simulink model "mrefrobotarm_modified_previous_y_previous_u_previous_ref_pert"  (R2018b)
settings: Solver=FixedStepAuto  StartTime=0.0  StopTime=10  RelTol=1e-3  AbsTol=1e-6
undefined symbols (not defined in the file or in its folder): cc, options
libraries: neural x714, simulink x1
(part 20 of 26)

== system mrefrobotarm_modified_previous_y_previous_u_previous_ref_pert/sd=0.1/Layer 3/Delays 1 ==
  "p{3}" : Inport  PortDimensions=30
      mask Display: e = 0.06;c1 = [120 230 180]/255;c2 = ([120 230 180]+0)/(256+128);c3 = ([120 230 180]+128)/(256+128);patch([0 1 1 0],[0 0 1 1],c1);patch([0 1 1 1-e 1-e 0+e],[0 0 1 1-e 0+e 0+e],c2);patch([0 0 1 1-e 0+e 0+e],[0 1 1 1-e 1-e 0+e],c3);plot([0 1 1 0 0],[0 0 1 1 0]);
  mux : Mux  Inputs=1
      mask Display: e = 0.06;c1 = [120 150 230]/255;c2 = ([120 150 230]+0)/383;c3 = ([120 150 230]+128)/383;patch([0 1 1 0],[0 0 1 1],c1);patch([0 1 1 1-e 1-e 0+e],[0 0 1 1-e 0+e 0+e],c2);patch([0 0 1 1-e 0+e 0+e],[0 1 1 1-e 1-e 0+e],c3);plot([0 1 1 0 0],[0 0 1 1 0]);disp('Mux')
  "pd{3,2}" : Outport
      mask Display: e = 0.06;c1 = [120 230 180]/255;c2 = ([120 230 180]+0)/(256+128);c3 = ([120 230 180]+128)/(256+128);patch([0 1 1 0],[0 0 1 1],c1);patch([0 1 1 1-e 1-e 0+e],[0 0 1 1-e 0+e 0+e],c2);patch([0 0 1 1-e 0+e 0+e],[0 1 1 1-e 1-e 0+e],c3);plot([0 1 1 0 0],[0 0 1 1 0]);
  wires:
  "p{3}"/1 -> mux/1
  mux/1 -> "pd{3,2}"/1

== system mrefrobotarm_modified_previous_y_previous_u_previous_ref_pert/sd=0.1/Layer 3/LW{3,2} ==
  "ad{3,2}" : Inport  PortDimensions=30
      mask Display: e = 0.06;c1 = [120 230 180]/255;c2 = ([120 230 180]+0)/(256+128);c3 = ([120 230 180]+128)/(256+128);patch([0 1 1 0],[0 0 1 1],c1);patch([0 1 1 1-e 1-e 0+e],[0 0 1 1-e 0+e 0+e],c2);patch([0 0 1 1-e 0+e 0+e],[0 1 1 1-e 1-e 0+e],c3);plot([0 1 1 0 0],[0 0 1 1 0]);
  "IW{3,2}(1,:)'" : Constant  Value=[0.0018188839666211098489156938740052282810211181640625;-0.0126510816907239136142049318323188344947993755340576171875;-0.00597472431956966830435273863031397922895848751068115234375;0.005949992205404812384283985693400609306991100311279296875;-0.018958893167521397027375229527024202980101108551025390625;-0.007711057222642365809039954882564416038803756237030029296875;-0.010778308261510882726241788986953906714916229248046875;0.054764058581412124182552503270926536060869693756103515625;0.006862056331544587849113892019659033394418656826019287109375;0.00715707547253511232321354640362187637947499752044677734375;-0.0016983245624861524614157559653904172591865062713623046875;-0.0065973873363838371475242894348411937244236469268798828125;-0.037341973875675053828881999606892350129783153533935546875;0.0018086616996149107450264637009240686893463134765625;-0.00260391987922085899054280844211461953818798065185546875;-0.0307949849301379675881040753893103101290762424468994140625;0.0170954132041403715491778569912639795802533626556396484375;-0.00466213820726418988471539961437883903272449970245361328125;0.004629973795378283969725874413825295050628483295440673828125;-0.0119610632763333425698792922275970340706408023834228515625;-0.01430710633569359270522713956097504706121981143951416015625;-0.033746901411126815906182940807411796413362026214599609375;0.50788162427434002665904699824750423431396484375;0.0104845825353180772954164723387293634004890918731689453125;-0.0039154731651121210678212491984595544636249542236328125;0.00908007893074675755118452258329853066243231296539306640625;0.004049068749268728943657702501468520495109260082244873046875;-0.0007508777613577442659742455788318693521432578563690185546875;-0.002722985317096936197511780619606724940240383148193359375;0.002330981056152135223735744062878438853658735752105712890625]
      mask Display: e = 0.06;c1 = [120 150 230]/255;c2 = ([120 150 230]+0)/383;c3 = ([120 150 230]+128)/383;patch([0 1 1 0],[0 0 1 1],c1);patch([0 1 1 1-e 1-e 0+e],[0 0 1 1-e 0+e 0+e],c2);patch([0 0 1 1-e 0+e 0+e],[0 1 1 1-e 1-e 0+e],c3);plot([0 1 1 0 0],[0 0 1 1 0]);disp('weights');
  Mux : Mux  Inputs=1
      mask Display: e = 0.06;c1 = [120 150 230]/255;c2 = ([120 150 230]+0)/383;c3 = ([120 150 230]+128)/383;patch([0 1 1 0],[0 0 1 1],c1);patch([0 1 1 1-e 1-e 0+e],[0 0 1 1-e 0+e 0+e],c2);patch([0 0 1 1-e 0+e 0+e],[0 1 1 1-e 1-e 0+e],c3);plot([0 1 1 0 0],[0 0 1 1 0]);disp('Mux');
  dotprod1 : neural/Weight Functions/dotprod
  "lz{3,2}" : Outport
      mask Display: e = 0.06;c1 = [120 230 180]/255;c2 = ([120 230 180]+0)/(256+128);c3 = ([120 230 180]+128)/(256+128);patch([0 1 1 0],[0 0 1 1],c1);patch([0 1 1 1-e 1-e 0+e],[0 0 1 1-e 0+e 0+e],c2);patch([0 0 1 1-e 0+e 0+e],[0 1 1 1-e 1-e 0+e],c3);plot([0 1 1 0 0],[0 0 1 1 0]);
  wires:
  "IW{3,2}(1,:)'"/1 -> dotprod1/1
  "ad{3,2}"/1 -> dotprod1/2
  dotprod1/1 -> Mux/1
  Mux/1 -> "lz{3,2}"/1

== system mrefrobotarm_modified_previous_y_previous_u_previous_ref_pert/sd=0.2/Layer 1/Delays 1 ==
  "p{1}" : Inport  PortDimensions=10
      mask Display: e = 0.06;c1 = [120 230 180]/255;c2 = ([120 230 180]+0)/(256+128);c3 = ([120 230 180]+128)/(256+128);patch([0 1 1 0],[0 0 1 1],c1);patch([0 1 1 1-e 1-e 0+e],[0 0 1 1-e 0+e 0+e],c2);patch([0 0 1 1-e 0+e 0+e],[0 1 1 1-e 1-e 0+e],c3);plot([0 1 1 0 0],[0 0 1 1 0]);
  mux : Mux  Inputs=1
      mask Display: e = 0.06;c1 = [120 150 230]/255;c2 = ([120 150 230]+0)/383;c3 = ([120 150 230]+128)/383;patch([0 1 1 0],[0 0 1 1],c1);patch([0 1 1 1-e 1-e 0+e],[0 0 1 1-e 0+e 0+e],c2);patch([0 0 1 1-e 0+e 0+e],[0 1 1 1-e 1-e 0+e],c3);plot([0 1 1 0 0],[0 0 1 1 0]);disp('Mux')
  "pd{1,1}" : Outport
      mask Display: e = 0.06;c1 = [120 230 180]/255;c2 = ([120 230 180]+0)/(256+128);c3 = ([120 230 180]+128)/(256+128);patch([0 1 1 0],[0 0 1 1],c1);patch([0 1 1 1-e 1-e 0+e],[0 0 1 1-e 0+e 0+e],c2);patch([0 0 1 1-e 0+e 0+e],[0 1 1 1-e 1-e 0+e],c3);plot([0 1 1 0 0],[0 0 1 1 0]);
  wires:
  "p{1}"/1 -> mux/1
  mux/1 -> "pd{1,1}"/1

== system mrefrobotarm_modified_previous_y_previous_u_previous_ref_pert/sd=0.2/Layer 1/IW{1,1} ==
  "pd{1,1}" : Inport  PortDimensions=10
      mask Display: e = 0.06;c1 = [120 230 180]/255;c2 = ([120 230 180]+0)/(256+128);c3 = ([120 230 180]+128)/(256+128);patch([0 1 1 0],[0 0 1 1],c1);patch([0 1 1 1-e 1-e 0+e],[0 0 1 1-e 0+e 0+e],c2);patch([0 0 1 1-e 0+e 0+e],[0 1 1 1-e 1-e 0+e],c3);plot([0 1 1 0 0],[0 0 1 1 0]);
  "IW{1,1}(1,:)'" : Constant  Value=[0.51497279749678614990671121631748974323272705078125;1.206829650462811986955102838692255318164825439453125;-0.0843780927922921641926023994528804905712604522705078125;1.0983052451279047279086853450280614197254180908203125;1.826296411118257356775984590058214962482452392578125;-0.229783480998378475401722198512288741767406463623046875;0.44712104438269906214742377414950169622898101806640625;-0.342730536328451018679430717384093441069126129150390625;1.0259047401059024906544436817057430744171142578125;-0.2128168709740031749877431366257951594889163970947265625]
      mask Display: e = 0.06;c1 = [120 150 230]/255;c2 = ([120 150 230]+0)/383;c3 = ([120 150 230]+128)/383;patch([0 1 1 0],[0 0 1 1],c1);patch([0 1 1 1-e 1-e 0+e],[0 0 1 1-e 0+e 0+e],c2);patch([0 0 1 1-e 0+e 0+e],[0 1 1 1-e 1-e 0+e],c3);plot([0 1 1 0 0],[0 0 1 1 0]);disp('Weights');
  "IW{1,1}(10,:)'" : Constant  Value=[-0.290019837810844283154665390611626207828521728515625;1.202814314763049008405459971982054412364959716796875;0.64575006256269118498636316871852613985538482666015625;0.51228702422282612616299957153387367725372314453125;0.53897724154057058409961200595716945827007293701171875;0.2169804329551216770521904209090280346572399139404296875;1.109828612580184170610664295963943004608154296875;0.62047060970846767968822632610681466758251190185546875;0.701249951108816826916836362215690314769744873046875;-0.2409479446688067849624559357835096307098865509033203125]
      mask Display: e = 0.06;c1 = [120 150 230]/255;c2 = ([120 150 230]+0)/383;c3 = ([120 150 230]+128)/383;patch([0 1 1 0],[0 0 1 1],c1);patch([0 1 1 1-e 1-e 0+e],[0 0 1 1-e 0+e 0+e],c2);patch([0 0 1 1-e 0+e 0+e],[0 1 1 1-e 1-e 0+e],c3);plot([0 1 1 0 0],[0 0 1 1 0]);disp('Weights');
  "IW{1,1}(11,:)'" : Constant  Value=[-0.483965255554764939294187797713675536215305328369140625;-0.00423735713268407789000580265792450518347322940826416015625;-0.04071278147423264270887699467493803240358829498291015625;-0.063810707355427875864251063831034116446971893310546875;0.63945678291134344650714638191857375204563140869140625;-0.293214326660526103385251417421386577188968658447265625;-0.2489985904371469771501068635188858024775981903076171875;-0.243620889480985258757073097513057291507720947265625;0.89874278529941487025922697284840978682041168212890625;0.391843733467475308085425922399736009538173675537109375]
      mask Display: e = 0.06;c1 = [120 150 230]/255;c2 = ([120 150 230]+0)/383;c3 = ([120 150 230]+128)/383;patch([0 1 1 0],[0 0 1 1],c1);patch([0 1 1 1-e 1-e 0+e],[0 0 1 1-e 0+e 0+e],c2);patch([0 0 1 1-e 0+e 0+e],[0 1 1 1-e 1-e 0+e],c3);plot([0 1 1 0 0],[0 0 1 1 0]);disp('Weights');
  "IW{1,1}(12,:)'" : Constant  Value=[0.1612342900655281130450902082884567789733409881591796875;0.83783524521083052594150331060518510639667510986328125;-0.6105547643586188844011530818534083664417266845703125;0.93437549886920745478846583864651620388031005859375;-0.41271403386041505267911588816787116229534149169921875;-0.2038648125981606662460166035089059732854366302490234375;-0.79779908968110169187326619066880084574222564697265625;0.212892509754028680379889237883617170155048370361328125;1.613792336196116838920033842441625893115997314453125;-0.005932794346736929014252126535211573354899883270263671875]
      mask Display: e = 0.06;c1 = [120 150 230]/255;c2 = ([120 150 230]+0)/383;c3 = ([120 150 230]+128)/383;patch([0 1 1 0],[0 0 1 1],c1);patch([0 1 1 1-e 1-e 0+e],[0 0 1 1-e 0+e 0+e],c2);patch([0 0 1 1-e 0+e 0+e],[0 1 1 1-e 1-e 0+e],c3);plot([0 1 1 0 0],[0 0 1 1 0]);disp('Weights');
  "IW{1,1}(13,:)'" : Constant  Value=[-0.1362341877538358059229750551821780391037464141845703125;0.954572016628826958140052738599479198455810546875;1.4567774435177611724867574594100005924701690673828125;0.1398942982446665095341842288689804263412952423095703125;0.22521814577160992332238720337045378983020782470703125;0.94253660172752018464592538293800316751003265380859375;0.6447180725726564531896656262688338756561279296875;0.782760397215020109484839849756099283695220947265625;-0.755379723776314460081948709557764232158660888671875;0.7209229108371120187115366206853650510311126708984375]
      mask Display: e = 0.06;c1 = [120 150 230]/255;c2 = ([120 150 230]+0)/383;c3 = ([120 150 230]+128)/383;patch([0 1 1 0],[0 0 1 1],c1);patch([0 1 1 1-e 1-e 0+e],[0 0 1 1-e 0+e 0+e],c2);patch([0 0 1 1-e 0+e 0+e],[0 1 1 1-e 1-e 0+e],c3);plot([0 1 1 0 0],[0 0 1 1 0]);disp('Weights');
  "IW{1,1}(14,:)'" : Constant  Value=[0.3848296502569208410449164148303680121898651123046875;-0.0848479163709470185494865290820598602294921875;-0.06685187407183122709763978264163597486913204193115234375;-0.12513880958835532641870713632670231163501739501953125;0.803549161421274416028381892829202115535736083984375;-1.130139231574783575950959857436828315258026123046875;-0.191640285152762268605641793328686617314815521240234375;0.212885117495971110113117674700333736836910247802734375;1.0074860578633748620092092096456326544284820556640625;-0.5140243939426916153223601213539950549602508544921875]
      mask Display: e = 0.06;c1 = [120 150 230]/255;c2 = ([120 150 230]+0)/383;c3 = ([120 150 230]+128)/383;patch([0 1 1 0],[0 0 1 1],c1);patch([0 1 1 1-e 1-e 0+e],[0 0 1 1-e 0+e 0+e],c2);patch([0 0 1 1-e 0+e 0+e],[0 1 1 1-e 1-e 0+e],c3);plot([0 1 1 0 0],[0 0 1 1 0]);disp('Weights');
  "IW{1,1}(15,:)'" : Constant  Value=[0.50448118661232588255671771548804827034473419189453125;0.75534739506285131227514284546487033367156982421875;0.7186274496868938488347566817537881433963775634765625;1.1053410499284714862966438886360265314579010009765625;1.55113744248226215205477274139411747455596923828125;-0.84818341679632347496209376913611777126789093017578125;0.85626822715970429822363030325504951179027557373046875;1.0587139812572943231572253353078849613666534423828125;-1.3036773470877511815757543445215560495853424072265625;-0.2345687264122083004469487832466256804764270782470703125]
      mask Display: e = 0.06;c1 = [120 150 230]/255;c2 = ([120 150 230]+0)/383;c3 = ([120 150 230]+128)/383;patch([0 1 1 0],[0 0 1 1],c1);patch([0 1 1 1-e 1-e 0+e],[0 0 1 1-e 0+e 0+e],c2);patch([0 0 1 1-e 0+e 0+e],[0 1 1 1-e 1-e 0+e],c3);plot([0 1 1 0 0],[0 0 1 1 0]);disp('Weights');
  "IW{1,1}(16,:)'" : Constant  Value=[0.89365107384404296464452954751322977244853973388671875;-0.5783582377704370447446535763447172939777374267578125;0.420643159623975193550649009921471588313579559326171875;0.71330291898780273651681227420340292155742645263671875;-0.1639046914328597670529319429988390766084194183349609375;-0.6859259654691352015021266197436489164829254150390625;-0.61633315473276628626564388468977995216846466064453125;-0.092017477242366918499527628227951936423778533935546875;0.217597708674847734044988101231865584850311279296875;-0.79075863473493601674135788925923407077789306640625]
      mask Display: e = 0.06;c1 = [120 150 230]/255;c2 = ([120 150 230]+0)/383;c3 = ([120 150 230]+128)/383;patch([0 1 1 0],[0 0 1 1],c1);patch([0 1 1 1-e 1-e 0+e],[0 0 1 1-e 0+e 0+e],c2);patch([0 0 1 1-e 0+e 0+e],[0 1 1 1-e 1-e 0+e],c3);plot([0 1 1 0 0],[0 0 1 1 0]);disp('Weights');
  "IW{1,1}(17,:)'" : Constant  Value=[0.1749980365235693502423686140900827012956142425537109375;-0.7277784587097422264179158446495421230792999267578125;0.275945189206802055092992986828903667628765106201171875;-0.6392369514218396719940074035548605024814605712890625;-0.326500751272584321949210561797372065484523773193359375;-2.011658986992188591358399207820184528827667236328125;-0.419988809430309195658281851137871854007244110107421875;0.92813668878189281574719871059642173349857330322265625;1.21675385461894602912025220575742423534393310546875;0.2135955828125577771192666887145605869591236114501953125]
      mask Display: e = 0.06;c1 = [120 150 230]/255;c2 = ([120 150 230]+0)/383;c3 = ([120 150 230]+128)/383;patch([0 1 1 0],[0 0 1 1],c1);patch([0 1 1 1-e 1-e 0+e],[0 0 1 1-e 0+e 0+e],c2);patch([0 0 1 1-e 0+e 0+e],[0 1 1 1-e 1-e 0+e],c3);plot([0 1 1 0 0],[0 0 1 1 0]);disp('Weights');
  "IW{1,1}(18,:)'" : Constant  Value=[-0.70447743533780526892229545410373248159885406494140625;0.441077583618011026533878293776069767773151397705078125;-0.2840705583921272481262576548033393919467926025390625;-0.6114067892875996168555730037041939795017242431640625;-0.80768131804438103582555186221725307404994964599609375;-0.344685562123354161112587235038517974317073822021484375;0.80642821071720083292433400856680236756801605224609375;0.07920147803555976917522229996393434703350067138671875;0.220187399237146197439329853295930661261081695556640625;0.3401071901510046568972711611422710120677947998046875]
      mask Display: e = 0.06;c1 = [120 150 230]/255;c2 = ([120 150 230]+0)/383;c3 = ([120 150 230]+128)/383;patch([0 1 1 0],[0 0 1 1],c1);patch([0 1 1 1-e 1-e 0+e],[0 0 1 1-e 0+e 0+e],c2);patch([0 0 1 1-e 0+e 0+e],[0 1 1 1-e 1-e 0+e],c3);plot([0 1 1 0 0],[0 0 1 1 0]);disp('Weights');
  "IW{1,1}(19,:)'" : Constant  Value=[0.3365345950967177923729423127952031791210174560546875;-0.159705462963764366346453016376472078263759613037109375;-0.218737820896978185647441250694100745022296905517578125;-0.5859069458641685823607758720754645764827728271484375;-1.3530134122432997401119791902601718902587890625;1.5819145945145194342984495960990898311138153076171875;-0.1516391720362563477753070628750720061361789703369140625;0.1854431550039121467943203924733097665011882781982421875;-1.617497693422686122488585169776342809200286865234375;-0.2406780160488969644294598992928513325750827789306640625]
      mask Display: e = 0.06;c1 = [120 150 230]/255;c2 = ([120 150 230]+0)/383;c3 = ([120 150 230]+128)/383;patch([0 1 1 0],[0 0 1 1],c1);patch([0 1 1 1-e 1-e 0+e],[0 0 1 1-e 0+e 0+e],c2);patch([0 0 1 1-e 0+e 0+e],[0 1 1 1-e 1-e 0+e],c3);plot([0 1 1 0 0],[0 0 1 1 0]);disp('Weights');
  "IW{1,1}(2,:)'" : Constant  Value=[1.1735222907779581102971633299603126943111419677734375;-1.0340438082621934423599441288388334214687347412109375;-0.1294633900950683813579900061085936613380908966064453125;-0.981840755571067091977965901605784893035888671875;0.036597406073111009294773765532227116636931896209716796875;1.310116040467077080933222532621584832668304443359375;-0.11330354187896048145933747264280100353062152862548828125;-0.39198876636958923658227149644517339766025543212890625;0.0448891996045359953360076588069205172359943389892578125;-0.5434775071875737051385613085585646331310272216796875]
      mask Display: e = 0.06;c1 = [120 150 230]/255;c2 = ([120 150 230]+0)/383;c3 = ([120 150 230]+128)/383;patch([0 1 1 0],[0 0 1 1],c1);patch([0 1 1 1-e 1-e 0+e],[0 0 1 1-e 0+e 0+e],c2);patch([0 0 1 1-e 0+e 0+e],[0 1 1 1-e 1-e 0+e],c3);plot([0 1 1 0 0],[0 0 1 1 0]);disp('Weights');
  "IW{1,1}(20,:)'" : Constant  Value=[-0.49080796088417366629386151544167660176753997802734375;-0.32658115404625487343537315609864890575408935546875;-0.30715298358569909087378846379579044878482818603515625;-0.2376225765599234984737364584361785091459751129150390625;-0.70709582393641789987981383092119358479976654052734375;-0.83764094852303550009509081064607016742229461669921875;-0.346888838416566425149056840382399968802928924560546875;0.85989098342755043713481200029491446912288665771484375;-0.37521274590153208539078377725672908127307891845703125;1.12614413773067401081107163918204605579376220703125]
      mask Display: e = 0.06;c1 = [120 150 230]/255;c2 = ([120 150 230]+0)/383;c3 = ([120 150 230]+128)/383;patch([0 1 1 0],[0 0 1 1],c1);patch([0 1 1 1-e 1-e 0+e],[0 0 1 1-e 0+e 0+e],c2);patch([0 0 1 1-e 0+e 0+e],[0 1 1 1-e 1-e 0+e],c3);plot([0 1 1 0 0],[0 0 1 1 0]);disp('Weights');
  "IW{1,1}(3,:)'" : Constant  Value=[-0.81788029602188039302035349464858882129192352294921875;-1.7460377417644428188481242614216171205043792724609375;-0.344830252014250493441949174666660837829113006591796875;0.94191811500333832984921400566236115992069244384765625;0.560417176129761163139164636959321796894073486328125;-0.2243598139544523417665544684496126137673854827880859375;-0.541006371143894160269383064587600529193878173828125;-0.25151592947967615909732330692349933087825775146484375;0.03514726839770783428651412805265863426029682159423828125;0.6677731755213536235515903172199614346027374267578125]
      mask Display: e = 0.06;c1 = [120 150 230]/255;c2 = ([120 150 230]+0)/383;c3 = ([120 150 230]+128)/383;patch([0 1 1 0],[0 0 1 1],c1);patch([0 1 1 1-e 1-e 0+e],[0 0 1 1-e 0+e 0+e],c2);patch([0 0 1 1-e 0+e 0+e],[0 1 1 1-e 1-e 0+e],c3);plot([0 1 1 0 0],[0 0 1 1 0]);disp('Weights');
  "IW{1,1}(4,:)'" : Constant  Value=[-0.1893981806756664110213961293993634171783924102783203125;1.043075870297573093381515718647278845310211181640625;0.59532765310384572199353669930133037269115447998046875;0.2255183197984091114651761245113448239862918853759765625;0.78778782036779626540834442494087852537631988525390625;-0.50003889566063441929344435266102664172649383544921875;0.290042355773057369816569917020387947559356689453125;0.390495576369537966687772723162197507917881011962890625;-1.1423046352205921127875853926525451242923736572265625;-0.8666626587426637939870488480664789676666259765625]
      mask Display: e = 0.06;c1 = [120 150 230]/255;c2 = ([120 150 230]+0)/383;c3 = ([120 150 230]+128)/383;patch([0 1 1 0],[0 0 1 1],c1);patch([0 1 1 1-e 1-e 0+e],[0 0 1 1-e 0+e 0+e],c2);patch([0 0 1 1-e 0+e 0+e],[0 1 1 1-e 1-e 0+e],c3);plot([0 1 1 0 0],[0 0 1 1 0]);disp('Weights');
  "IW{1,1}(5,:)'" : Constant  Value=[0.98526687568134219130655537810525856912136077880859375;-0.26998052201425937202117211199947632849216461181640625;0.00499871613682153874413938154930292512290179729461669921875;0.295223917912018907205862205955781973898410797119140625;0.0967245625040197565258637268925667740404605865478515625;0.1020661850288483163406993980970582924783229827880859375;-1.1233460342285568334119716382701881229877471923828125;-0.264901944476280404305867932635010220110416412353515625;-1.1915924020027552909795076629961840808391571044921875;-0.781434341043083069422436892637051641941070556640625]
      mask Display: e = 0.06;c1 = [120 150 230]/255;c2 = ([120 150 230]+0)/383;c3 = ([120 150 230]+128)/383;patch([0 1 1 0],[0 0 1 1],c1);patch([0 1 1 1-e 1-e 0+e],[0 0 1 1-e 0+e 0+e],c2);patch([0 0 1 1-e 0+e 0+e],[0 1 1 1-e 1-e 0+e],c3);plot([0 1 1 0 0],[0 0 1 1 0]);disp('Weights');
  "IW{1,1}(6,:)'" : Constant  Value=[0.1420691339825521926076845602437970228493213653564453125;0.6263202631863205027684671222232282161712646484375;0.8107642320241381650447465290199033915996551513671875;-0.9432080474995874208588020337629131972789764404296875;-0.95030083307769641631779222734621725976467132568359375;-0.6484915591630515674381740609533153474330902099609375;-0.312936741608584256812974899730761535465717315673828125;0.88487981709345520098253246032982133328914642333984375;0.4628411150217506264681333050248213112354278564453125;-1.2230325970732665030737962297280319035053253173828125]
      mask Display: e = 0.06;c1 = [120 150 230]/255;c2 = ([120 150 230]+0)/383;c3 = ([120 150 230]+128)/383;patch([0 1 1 0],[0 0 1 1],c1);patch([0 1 1 1-e 1-e 0+e],[0 0 1 1-e 0+e 0+e],c2);patch([0 0 1 1-e 0+e 0+e],[0 1 1 1-e 1-e 0+e],c3);plot([0 1 1 0 0],[0 0 1 1 0]);disp('Weights');
  "IW{1,1}(7,:)'" : Constant  Value=[-0.500648315412738131868763957754708826541900634765625;-0.95983765310247870505833134302520193159580230712890625;-0.5217048267007278194995478770579211413860321044921875;-0.43075548922962081377363574574701488018035888671875;0.7141696229922509520093854007427580654621124267578125;-0.70200098378879172145161646767519414424896240234375;0.60244783079223329647078344351029954850673675537109375;-0.38737653697134855068640035824500955641269683837890625;-0.79492311138001314763101845528581179678440093994140625;-0.6211610951181081308192233336740173399448394775390625]
      mask Display: e = 0.06;c1 = [120 150 230]/255;c2 = ([120 150 230]+0)/383;c3 = ([120 150 230]+128)/383;patch([0 1 1 0],[0 0 1 1],c1);patch([0 1 1 1-e 1-e 0+e],[0 0 1 1-e 0+e 0+e],c2);patch([0 0 1 1-e 0+e 0+e],[0 1 1 1-e 1-e 0+e],c3);plot([0 1 1 0 0],[0 0 1 1 0]);disp('Weights');
  "IW{1,1}(8,:)'" : Constant  Value=[-0.493719289839638919570319330887286923825740814208984375;0.36147487297337244083195173516287468373775482177734375;-0.4321415122307230571863101431517861783504486083984375;-0.37897843791982033234688742595608346164226531982421875;-1.5350878964443144258922302469727583229541778564453125;0.210809893287703165043467379291541874408721923828125;0.191911403926806445330299766283133067190647125244140625;0.3565449447961308582222272889339365065097808837890625;-0.61639660811120677852414928565849550068378448486328125;-0.08778370961064474453650063878740184009075164794921875]
      mask Display: e = 0.06;c1 = [120 150 230]/255;c2 = ([120 150 230]+0)/383;c3 = ([120 150 230]+128)/383;patch([0 1 1 0],[0 0 1 1],c1);patch([0 1 1 1-e 1-e 0+e],[0 0 1 1-e 0+e 0+e],c2);patch([0 0 1 1-e 0+e 0+e],[0 1 1 1-e 1-e 0+e],c3);plot([0 1 1 0 0],[0 0 1 1 0]);disp('Weights');
  "IW{1,1}(9,:)'" : Constant  Value=[1.3293314592685707697938823912409134209156036376953125;0.222838342886467588588317312314757145941257476806640625;-0.92463328047312398627610718904179520905017852783203125;0.63925523648537596610452737877494655549526214599609375;-0.89514742868651620000264301779679954051971435546875;0.075940422453930678248212871039868332445621490478515625;-1.148250497395655767007838221616111695766448974609375;-0.13710946150061775750117476491141133010387420654296875;0.3608958290886394859597885442781262099742889404296875;0.495407140859233041663145513666677288711071014404296875]
      mask Display: e = 0.06;c1 = [120 150 230]/255;c2 = ([120 150 230]+0)/383;c3 = ([120 150 230]+128)/383;patch([0 1 1 0],[0 0 1 1],c1);patch([0 1 1 1-e 1-e 0+e],[0 0 1 1-e 0+e 0+e],c2);patch([0 0 1 1-e 0+e 0+e],[0 1 1 1-e 1-e 0+e],c3);plot([0 1 1 0 0],[0 0 1 1 0]);disp('Weights');
  Mux : Mux  Inputs=20
      mask Display: e = 0.06;c1 = [120 150 230]/255;c2 = ([120 150 230]+0)/383;c3 = ([120 150 230]+128)/383;patch([0 1 1 0],[0 0 1 1],c1);patch([0 1 1 1-e 1-e 0+e],[0 0 1 1-e 0+e 0+e],c2);patch([0 0 1 1-e 0+e 0+e],[0 1 1 1-e 1-e 0+e],c3);plot([0 1 1 0 0],[0 0 1 1 0]);disp('Mux');
  dotprod{1..20} (20 alike) : neural/Weight Functions/dotprod
  "iz{1,1}" : Outport
      mask Display: e = 0.06;c1 = [120 230 180]/255;c2 = ([120 230 180]+0)/(256+128);c3 = ([120 230 180]+128)/(256+128);patch([0 1 1 0],[0 0 1 1],c1);patch([0 1 1 1-e 1-e 0+e],[0 0 1 1-e 0+e 0+e],c2);patch([0 0 1 1-e 0+e 0+e],[0 1 1 1-e 1-e 0+e],c3);plot([0 1 1 0 0],[0 0 1 1 0]);
  wires:
  "IW{1,1}(1,:)'"/1 -> dotprod1/1
  "pd{1,1}"/1 -> dotprod1/2, dotprod2/2, dotprod3/2, dotprod4/2, dotprod5/2, dotprod6/2, dotprod7/2, dotprod8/2, dotprod9/2, dotprod10/2, dotprod11/2, dotprod12/2, dotprod13/2, dotprod14/2, dotprod15/2, dotprod16/2, dotprod17/2, dotprod18/2, dotprod19/2, dotprod20/2
  dotprod1/1 -> Mux/1
  "IW{1,1}(2,:)'"/1 -> dotprod2/1
  dotprod2/1 -> Mux/2
  "IW{1,1}(3,:)'"/1 -> dotprod3/1
  dotprod3/1 -> Mux/3
  "IW{1,1}(4,:)'"/1 -> dotprod4/1
  dotprod4/1 -> Mux/4
  "IW{1,1}(5,:)'"/1 -> dotprod5/1
  dotprod5/1 -> Mux/5
  "IW{1,1}(6,:)'"/1 -> dotprod6/1
  dotprod6/1 -> Mux/6
  "IW{1,1}(7,:)'"/1 -> dotprod7/1
  dotprod7/1 -> Mux/7
  "IW{1,1}(8,:)'"/1 -> dotprod8/1
  dotprod8/1 -> Mux/8
  "IW{1,1}(9,:)'"/1 -> dotprod9/1
  dotprod9/1 -> Mux/9
  "IW{1,1}(10,:)'"/1 -> dotprod10/1
  dotprod10/1 -> Mux/10
  "IW{1,1}(11,:)'"/1 -> dotprod11/1
  dotprod11/1 -> Mux/11
  "IW{1,1}(12,:)'"/1 -> dotprod12/1
  dotprod12/1 -> Mux/12
  "IW{1,1}(13,:)'"/1 -> dotprod13/1
  dotprod13/1 -> Mux/13
  "IW{1,1}(14,:)'"/1 -> dotprod14/1
  dotprod14/1 -> Mux/14
  "IW{1,1}(15,:)'"/1 -> dotprod15/1
  dotprod15/1 -> Mux/15
  "IW{1,1}(16,:)'"/1 -> dotprod16/1
  dotprod16/1 -> Mux/16
  "IW{1,1}(17,:)'"/1 -> dotprod17/1
  dotprod17/1 -> Mux/17
  "IW{1,1}(18,:)'"/1 -> dotprod18/1
  dotprod18/1 -> Mux/18
  "IW{1,1}(19,:)'"/1 -> dotprod19/1
  dotprod19/1 -> Mux/19
  "IW{1,1}(20,:)'"/1 -> dotprod20/1
  dotprod20/1 -> Mux/20
  Mux/1 -> "iz{1,1}"/1

== system mrefrobotarm_modified_previous_y_previous_u_previous_ref_pert/sd=0.2/Layer 2/Delays 1 ==
  "p{2}" : Inport  PortDimensions=20
      mask Display: e = 0.06;c1 = [120 230 180]/255;c2 = ([120 230 180]+0)/(256+128);c3 = ([120 230 180]+128)/(256+128);patch([0 1 1 0],[0 0 1 1],c1);patch([0 1 1 1-e 1-e 0+e],[0 0 1 1-e 0+e 0+e],c2);patch([0 0 1 1-e 0+e 0+e],[0 1 1 1-e 1-e 0+e],c3);plot([0 1 1 0 0],[0 0 1 1 0]);
  mux : Mux  Inputs=1
      mask Display: e = 0.06;c1 = [120 150 230]/255;c2 = ([120 150 230]+0)/383;c3 = ([120 150 230]+128)/383;patch([0 1 1 0],[0 0 1 1],c1);patch([0 1 1 1-e 1-e 0+e],[0 0 1 1-e 0+e 0+e],c2);patch([0 0 1 1-e 0+e 0+e],[0 1 1 1-e 1-e 0+e],c3);plot([0 1 1 0 0],[0 0 1 1 0]);disp('Mux')
  "pd{2,1}" : Outport
      mask Display: e = 0.06;c1 = [120 230 180]/255;c2 = ([120 230 180]+0)/(256+128);c3 = ([120 230 180]+128)/(256+128);patch([0 1 1 0],[0 0 1 1],c1);patch([0 1 1 1-e 1-e 0+e],[0 0 1 1-e 0+e 0+e],c2);patch([0 0 1 1-e 0+e 0+e],[0 1 1 1-e 1-e 0+e],c3);plot([0 1 1 0 0],[0 0 1 1 0]);
  wires:
  "p{2}"/1 -> mux/1
  mux/1 -> "pd{2,1}"/1

== system mrefrobotarm_modified_previous_y_previous_u_previous_ref_pert/sd=0.2/Layer 2/LW{2,1} ==
  "ad{2,1}" : Inport  PortDimensions=20
      mask Display: e = 0.06;c1 = [120 230 180]/255;c2 = ([120 230 180]+0)/(256+128);c3 = ([120 230 180]+128)/(256+128);patch([0 1 1 0],[0 0 1 1],c1);patch([0 1 1 1-e 1-e 0+e],[0 0 1 1-e 0+e 0+e],c2);patch([0 0 1 1-e 0+e 0+e],[0 1 1 1-e 1-e 0+e],c3);plot([0 1 1 0 0],[0 0 1 1 0]);
  "IW{2,1}(1,:)'" : Constant  Value=[0.76496661057361647895191936186165548861026763916015625;0.40082870222786437519602031898102723062038421630859375;0.6625793217714959215669523473479785025119781494140625;-0.282094746547580987883208081257180310785770416259765625;-0.67279574284390541993872147941146977245807647705078125;-0.041135386431857469402562088589547784067690372467041015625;-0.66436660930165114535839165910147130489349365234375;0.0965209242525334742968112777816713787615299224853515625;0.892552374657073155361786120920442044734954833984375;-0.5231358159442274224915081504150293767452239990234375;0.37607829500332534689022168095107190310955047607421875;-0.5928898185505782070237046355032362043857574462890625;0.59553730771049850911680323406471870839595794677734375;0.29513187862141443407182350711082108318805694580078125;0.637660057963431281535804373561404645442962646484375;0.08898568653668538497303330814247601665556430816650390625;-0.17669110219003825168471166762174107134342193603515625;0.329211328730071084436303863185457885265350341796875;0.49325934328156983976754190734936855733394622802734375;-0.0705846312106322149038106772422906942665576934814453125]
      mask Display: e = 0.06;c1 = [120 150 230]/255;c2 = ([120 150 230]+0)/383;c3 = ([120 150 230]+128)/383;patch([0 1 1 0],[0 0 1 1],c1);patch([0 1 1 1-e 1-e 0+e],[0 0 1 1-e 0+e 0+e],c2);patch([0 0 1 1-e 0+e 0+e],[0 1 1 1-e 1-e 0+e],c3);plot([0 1 1 0 0],[0 0 1 1 0]);disp('weights');
  "IW{2,1}(10,:)'" : Constant  Value=[0.0279378169814974430806842065067030489444732666015625;0.46967423642420158547139408256043680012226104736328125;0.238491853975729195536104043640079908072948455810546875;-0.0192540516848885741307828567414617282338440418243408203125;0.097501357869920035614796915979241020977497100830078125;0.478305839653533404476348778189276345074176788330078125;0.417893925120314702059687306245905347168445587158203125;-0.1320338790572588016924981957345153205096721649169921875;0.21628018481258071137318665932980366051197052001953125;-0.1556015449463256372641950520119280554354190826416015625;0.08074184783822803412878243989325710572302341461181640625;-0.307063446088555291879629294271580874919891357421875;0.245692090146631236802221565085346810519695281982421875;-0.565900161832816106510790632455609738826751708984375;0.355232831296197593129448932813829742372035980224609375;0.2374077413427641836118908713615383021533489227294921875;-0.00425767228843254054437839073443683446384966373443603515625;-0.1337082378528946791096387869401951320469379425048828125;0.043566557903260194617445222320384345948696136474609375;0.03944775832969800444249841575583559460937976837158203125]
      mask Display: e = 0.06;c1 = [120 150 230]/255;c2 = ([120 150 230]+0)/383;c3 = ([120 150 230]+128)/383;patch([0 1 1 0],[0 0 1 1],c1);patch([0 1 1 1-e 1-e 0+e],[0 0 1 1-e 0+e 0+e],c2);patch([0 0 1 1-e 0+e 0+e],[0 1 1 1-e 1-e 0+e],c3);plot([0 1 1 0 0],[0 0 1 1 0]);disp('weights');
  "IW{2,1}(2,:)'" : Constant  Value=[0.48099366495409945354566616515512578189373016357421875;0.0120773839077013799003790239794398075900971889495849609375;0.27322972584358506953350342882913537323474884033203125;-0.454162787590592476050233017303980886936187744140625;0.289803876110632130380651005907566286623477935791015625;-0.62204162038444243965074065272347070276737213134765625;-0.1846144040941755382068123481076327152550220489501953125;0.225582379404204946826695277195540256798267364501953125;-0.10825266679514744527779157579061575233936309814453125;0.331660315705087971327458262749132700264453887939453125;-1.1741596849901785315495317263412289321422576904296875;-0.56472914900433968110604610046721063554286956787109375;0.429585609882884467136676676091155968606472015380859375;0.121160024462371340714383904924034141004085540771484375;0.6405631919026208986878145879018120467662811279296875;0.438631305024265116809800701958010904490947723388671875;0.33389061474288028730228461427032016217708587646484375;0.25589807375190198879266745279892347753047943115234375;-0.0628121428650447455321881307099829427897930145263671875;-0.006618875516632199453026519364584601134993135929107666015625]
      mask Display: e = 0.06;c1 = [120 150 230]/255;c2 = ([120 150 230]+0)/383;c3 = ([120 150 230]+128)/383;patch([0 1 1 0],[0 0 1 1],c1);patch([0 1 1 1-e 1-e 0+e],[0 0 1 1-e 0+e 0+e],c2);patch([0 0 1 1-e 0+e 0+e],[0 1 1 1-e 1-e 0+e],c3);plot([0 1 1 0 0],[0 0 1 1 0]);disp('weights');
  "IW{2,1}(3,:)'" : Constant  Value=[-0.56438841797695038504656395161873660981655120849609375;-0.57911862846637396362581284847692586481571197509765625;-0.66292490903369183374849171741516329348087310791015625;-0.80280173104449115140113235611352138221263885498046875;-0.597130774059107860551876001409254968166351318359375;-0.3951021772913543284033721647574566304683685302734375;-0.8597797363556995975386598729528486728668212890625;-0.52939882422503259373769424200872890651226043701171875;-0.12072888324242081470316634295159019529819488525390625;-0.57769119490305598230150962990592233836650848388671875;-0.6433074127929341301523891161195933818817138671875;0.197315978864825825045414831038215197622776031494140625;-0.446740909313351586273910243107820861041545867919921875;-0.10139482703229631133101662499029771424829959869384765625;-0.515569253998520604653776899795047938823699951171875;-0.11226255699291219636304361984002753160893917083740234375;-0.46695740167935839703972078496008180081844329833984375;0.0288768947019422510258390701665121014229953289031982421875;0.2262210474124260184414225705040735192596912384033203125;0.175022956532774942584040900328545831143856048583984375]
      mask Display: e = 0.06;c1 = [120 150 230]/255;c2 = ([120 150 230]+0)/383;c3 = ([120 150 230]+128)/383;patch([0 1 1 0],[0 0 1 1],c1);patch([0 1 1 1-e 1-e 0+e],[0 0 1 1-e 0+e 0+e],c2);patch([0 0 1 1-e 0+e 0+e],[0 1 1 1-e 1-e 0+e],c3);plot([0 1 1 0 0],[0 0 1 1 0]);disp('weights');
  "IW{2,1}(4,:)'" : Constant  Value=[0.0523230775686112370426172901716199703514575958251953125;-0.811876936204331212110218984889797866344451904296875;-0.0183968618619299272010092494156197062693536281585693359375;-0.1476219902444679821229556182515807449817657470703125;0.1804846188910828874707448221670347265899181365966796875;0.020305322884345354539359362888717441819608211517333984375;-0.1326827073696405234759509994546533562242984771728515625;0.66409597043396517701552284052013419568538665771484375;-0.01765936787466181046024615852729766629636287689208984375;0.180923577607755070584261147814686410129070281982421875;-0.287497056419126317816647997460677288472652435302734375;0.1520479748823736210194823570418520830571651458740234375;-0.0651976496296517160633499088362441398203372955322265625;0.1144075850875492517122467006629449315369129180908203125;-0.319345872439719846713757078759954310953617095947265625;0.40006463073001696795216730606625787913799285888671875;-0.47067551135411722640355947078205645084381103515625;0.489519243933828895887216958726639859378337860107421875;0.63948711030027116652973973032203502953052520751953125;0.2487108992835832810275320525761344470083713531494140625]
      mask Display: e = 0.06;c1 = [120 150 230]/255;c2 = ([120 150 230]+0)/383;c3 = ([120 150 230]+128)/383;patch([0 1 1 0],[0 0 1 1],c1);patch([0 1 1 1-e 1-e 0+e],[0 0 1 1-e 0+e 0+e],c2);patch([0 0 1 1-e 0+e 0+e],[0 1 1 1-e 1-e 0+e],c3);plot([0 1 1 0 0],[0 0 1 1 0]);disp('weights');
  "IW{2,1}(5,:)'" : Constant  Value=[-0.35008483293397840707683599248412065207958221435546875;0.2296570620451217903390528363161138258874416351318359375;-0.01233460814728719844024507068525053909979760646820068359375;-0.1123322363673745771794898473672219552099704742431640625;0.5556649122241250626785813437891192734241485595703125;0.63745801805068025291944877608329989016056060791015625;-0.2380868453502480164285515229494194500148296356201171875;-0.08595421067440330020748007200381834991276264190673828125;-0.223097905870325796673370177813922055065631866455078125;0.193600174797834256867901103760232217609882354736328125;0.291884783006868875343542413247632794082164764404296875;0.1232144380272985062507729026037850417196750640869140625;0.1313755073149590890668747533709392882883548736572265625;0.52647770718378994470043608089326880872249603271484375;0.262601681051343682771204157688771374523639678955078125;0.1261723491455599421851019314999575726687908172607421875;-0.358501789007869609005041411364800296723842620849609375;0.219003083066970638537185323002631776034832000732421875;-0.64408858027657955869216266364674083888530731201171875;0.184958038297143578798653607009327970445156097412109375]
      mask Display: e = 0.06;c1 = [120 150 230]/255;c2 = ([120 150 230]+0)/383;c3 = ([120 150 230]+128)/383;patch([0 1 1 0],[0 0 1 1],c1);patch([0 1 1 1-e 1-e 0+e],[0 0 1 1-e 0+e 0+e],c2);patch([0 0 1 1-e 0+e 0+e],[0 1 1 1-e 1-e 0+e],c3);plot([0 1 1 0 0],[0 0 1 1 0]);disp('weights');
  "IW{2,1}(6,:)'" : Constant  Value=[0.0729620649957481715031093472134671173989772796630859375;-0.9945630756354797430418557269149459898471832275390625;0.4824264824251514038877530765603296458721160888671875;-0.10754256398773996694639976112739532254636287689208984375;0.2217045228975730031262258989954716525971889495849609375;-0.48839513868887463043932939399383030831813812255859375;0.66882977917390451505497139805811457335948944091796875;-0.56796515054863971894150154184899292886257171630859375;0.0136467358833525058414704034248643438331782817840576171875;-0.09997499273598296765097614979822537861764430999755859375;-0.27658560133933374203252242296002805233001708984375;-0.374453729719119554619766176983830519020557403564453125;-0.495199954770134898041078486130572855472564697265625;0.66859522473757759808421496927621774375438690185546875;-0.8368917256092771594921941868960857391357421875;-0.27828230743749049480584289995022118091583251953125;-0.7338513975986968862486037323833443224430084228515625;0.51195395306187208017689727057586424052715301513671875;0.02330340705918033938903732860126183368265628814697265625;0.06109010634619756185959005279073608107864856719970703125]
      mask Display: e = 0.06;c1 = [120 150 230]/255;c2 = ([120 150 230]+0)/383;c3 = ([120 150 230]+128)/383;patch([0 1 1 0],[0 0 1 1],c1);patch([0 1 1 1-e 1-e 0+e],[0 0 1 1-e 0+e 0+e],c2);patch([0 0 1 1-e 0+e 0+e],[0 1 1 1-e 1-e 0+e],c3);plot([0 1 1 0 0],[0 0 1 1 0]);disp('weights');
  "IW{2,1}(7,:)'" : Constant  Value=[0.47798140139116984670408783131279051303863525390625;0.45401025257122429312772737830528058111667633056640625;0.512035868790095438640719294198788702487945556640625;-0.525082253204666837831382508738897740840911865234375;-0.38103384501559656172275936114601790904998779296875;-0.3289311057449120223594718481763266026973724365234375;0.55100911424882215161602516673156060278415679931640625;0.501610164769443311882923808298073709011077880859375;-0.42802699133937960329632232969743199646472930908203125;-0.64255651883870423812794570039841346442699432373046875;0.956781716544366389598508249036967754364013671875;0.56231837191209044224393664990202523767948150634765625;-0.380049892393296173676020544007769785821437835693359375;-0.2367844430389414445148332788448897190392017364501953125;-0.431034057486032351480531588094891048967838287353515625;0.165960909726593552893092464728397317230701446533203125;0.471719725471719086851152269446174614131450653076171875;0.060245775536994672361146285766153596341609954833984375;-0.497017044806821350899639355702674947679042816162109375;0.605328809828616254407052110764198005199432373046875]
      mask Display: e = 0.06;c1 = [120 150 230]/255;c2 = ([120 150 230]+0)/383;c3 = ([120 150 230]+128)/383;patch([0 1 1 0],[0 0 1 1],c1);patch([0 1 1 1-e 1-e 0+e],[0 0 1 1-e 0+e 0+e],c2);patch([0 0 1 1-e 0+e 0+e],[0 1 1 1-e 1-e 0+e],c3);plot([0 1 1 0 0],[0 0 1 1 0]);disp('weights');
  "IW{2,1}(8,:)'" : Constant  Value=[-0.8287540601431455655756508349440991878509521484375;0.5742855246153586445956307215965352952480316162109375;-0.029412090151031043683271803956813528202474117279052734375;-0.90221269148091198797345668936031870543956756591796875;0.007060759256209560297268268413972691632807254791259765625;0.89593041532936457116420569946058094501495361328125;-0.244190342502142276881471616434282623231410980224609375;-0.88740217456005410223696117100189439952373504638671875;0.379260613477142627392169060840387828648090362548828125;-0.1669991270302168262507080953582772053778171539306640625;-0.69876333981533977901534626653301529586315155029296875;-0.7652653373649542789536326381494291126728057861328125;-0.28317345232264867771476701818755827844142913818359375;-1.4488327960538438521354009935748763382434844970703125;-0.1126121475710012143078841972965165041387081146240234375;0.420734563419441098819362423455459065735340118408203125;0.332831793691219568476213908070349134504795074462890625;0.49934774881148513703266189622809179127216339111328125;-0.6946993864425976550336372383753769099712371826171875;-0.2405724311936687787039090835605747997760772705078125]
      mask Display: e = 0.06;c1 = [120 150 230]/255;c2 = ([120 150 230]+0)/383;c3 = ([120 150 230]+128)/383;patch([0 1 1 0],[0 0 1 1],c1);patch([0 1 1 1-e 1-e 0+e],[0 0 1 1-e 0+e 0+e],c2);patch([0 0 1 1-e 0+e 0+e],[0 1 1 1-e 1-e 0+e],c3);plot([0 1 1 0 0],[0 0 1 1 0]);disp('weights');
  "IW{2,1}(9,:)'" : Constant  Value=[-0.345139253330120687746074281676555983722209930419921875;-0.436042228499868012026041697026812471449375152587890625;-0.1318777368243748415732596868110704235732555389404296875;-0.068184958659323446905631271874881349503993988037109375;-0.98966039181008458314181552850641310214996337890625;0.141778805510221317387475892246584407985210418701171875;1.4204087468472235133987169319880194962024688720703125;-0.73446417704829591865944848905201070010662078857421875;-0.56104934584132848396365034204791299998760223388671875;0.64773930363637022278311405898421071469783782958984375;0.75301183146501349252588397575891576707363128662109375;0.219186142949713114180809725439758040010929107666015625;0.065128614561248021619377368551795370876789093017578125;-0.187188666006862458601744947372935712337493896484375;-0.4224358950898887687941396507085300981998443603515625;0.1295823468069046413564393560591270215809345245361328125;0.2070658831614886341565551219900953583419322967529296875;0.1767955434682948190339146776750567369163036346435546875;1.2258647483244471398933228556415997445583343505859375;-0.321329194564977604908762032209779135882854461669921875]
      mask Display: e = 0.06;c1 = [120 150 230]/255;c2 = ([120 150 230]+0)/383;c3 = ([120 150 230]+128)/383;patch([0 1 1 0],[0 0 1 1],c1);patch([0 1 1 1-e 1-e 0+e],[0 0 1 1-e 0+e 0+e],c2);patch([0 0 1 1-e 0+e 0+e],[0 1 1 1-e 1-e 0+e],c3);plot([0 1 1 0 0],[0 0 1 1 0]);disp('weights');
  Mux : Mux  Inputs=10
      mask Display: e = 0.06;c1 = [120 150 230]/255;c2 = ([120 150 230]+0)/383;c3 = ([120 150 230]+128)/383;patch([0 1 1 0],[0 0 1 1],c1);patch([0 1 1 1-e 1-e 0+e],[0 0 1 1-e 0+e 0+e],c2);patch([0 0 1 1-e 0+e 0+e],[0 1 1 1-e 1-e 0+e],c3);plot([0 1 1 0 0],[0 0 1 1 0]);disp('Mux');
  dotprod{1..10} (10 alike) : neural/Weight Functions/dotprod
  "lz{2,1}" : Outport
      mask Display: e = 0.06;c1 = [120 230 180]/255;c2 = ([120 230 180]+0)/(256+128);c3 = ([120 230 180]+128)/(256+128);patch([0 1 1 0],[0 0 1 1],c1);patch([0 1 1 1-e 1-e 0+e],[0 0 1 1-e 0+e 0+e],c2);patch([0 0 1 1-e 0+e 0+e],[0 1 1 1-e 1-e 0+e],c3);plot([0 1 1 0 0],[0 0 1 1 0]);
  wires:
  "IW{2,1}(1,:)'"/1 -> dotprod1/1
  "ad{2,1}"/1 -> dotprod1/2, dotprod2/2, dotprod3/2, dotprod4/2, dotprod5/2, dotprod6/2, dotprod7/2, dotprod8/2, dotprod9/2, dotprod10/2
  dotprod1/1 -> Mux/1
  "IW{2,1}(2,:)'"/1 -> dotprod2/1
  dotprod2/1 -> Mux/2
  "IW{2,1}(3,:)'"/1 -> dotprod3/1
  dotprod3/1 -> Mux/3
  "IW{2,1}(4,:)'"/1 -> dotprod4/1
  dotprod4/1 -> Mux/4
  "IW{2,1}(5,:)'"/1 -> dotprod5/1
  dotprod5/1 -> Mux/5
  "IW{2,1}(6,:)'"/1 -> dotprod6/1
  dotprod6/1 -> Mux/6
  "IW{2,1}(7,:)'"/1 -> dotprod7/1
  dotprod7/1 -> Mux/7
  "IW{2,1}(8,:)'"/1 -> dotprod8/1
  dotprod8/1 -> Mux/8
  "IW{2,1}(9,:)'"/1 -> dotprod9/1
  dotprod9/1 -> Mux/9
  "IW{2,1}(10,:)'"/1 -> dotprod10/1
  dotprod10/1 -> Mux/10
  Mux/1 -> "lz{2,1}"/1

== system mrefrobotarm_modified_previous_y_previous_u_previous_ref_pert/sd=0.2/Layer 3/Delays 1 ==
  "p{3}" : Inport  PortDimensions=10
      mask Display: e = 0.06;c1 = [120 230 180]/255;c2 = ([120 230 180]+0)/(256+128);c3 = ([120 230 180]+128)/(256+128);patch([0 1 1 0],[0 0 1 1],c1);patch([0 1 1 1-e 1-e 0+e],[0 0 1 1-e 0+e 0+e],c2);patch([0 0 1 1-e 0+e 0+e],[0 1 1 1-e 1-e 0+e],c3);plot([0 1 1 0 0],[0 0 1 1 0]);
  mux : Mux  Inputs=1
      mask Display: e = 0.06;c1 = [120 150 230]/255;c2 = ([120 150 230]+0)/383;c3 = ([120 150 230]+128)/383;patch([0 1 1 0],[0 0 1 1],c1);patch([0 1 1 1-e 1-e 0+e],[0 0 1 1-e 0+e 0+e],c2);patch([0 0 1 1-e 0+e 0+e],[0 1 1 1-e 1-e 0+e],c3);plot([0 1 1 0 0],[0 0 1 1 0]);disp('Mux')
  "pd{3,2}" : Outport
      mask Display: e = 0.06;c1 = [120 230 180]/255;c2 = ([120 230 180]+0)/(256+128);c3 = ([120 230 180]+128)/(256+128);patch([0 1 1 0],[0 0 1 1],c1);patch([0 1 1 1-e 1-e 0+e],[0 0 1 1-e 0+e 0+e],c2);patch([0 0 1 1-e 0+e 0+e],[0 1 1 1-e 1-e 0+e],c3);plot([0 1 1 0 0],[0 0 1 1 0]);
  wires:
  "p{3}"/1 -> mux/1
  mux/1 -> "pd{3,2}"/1
